simulink model "ART_IDS_TUNING_SLDRT"  (R2021a)
settings: configuration reference "Normal_SLDRT" (kept outside this file)
undefined symbols (not defined in the file): channel, group_IP_address, receive_multicast_udp_port_initialize, release_receive_multicast_udp_buffer, TRDP_COM_ID_CCU2IDS, TRDP_COM_ID_MC1_IDS2CCU, TRDP_COM_ID_MC1_MMU2IDS_POINT, TRDP_COM_ID_MC1_MMU2IDS_SEGMENT, TRDP_COM_ID_MC2_IDS2CCU, TRDP_COM_ID_MC2_MMU2IDS_POINT, TRDP_COM_ID_MC2_MMU2IDS_SEGMENT, TRDP_CONFIG_MC1_CCU2IDS, TRDP_CONFIG_MC1_IDS2CCU, TRDP_CONFIG_MC1_MMU2IDS_POINT, TRDP_CONFIG_MC1_MMU2IDS_SEGMENT, TRDP_CONFIG_MC2_CCU2IDS, TRDP_CONFIG_MC2_IDS2CCU, TRDP_CONFIG_MC2_MMU2IDS_POINT, TRDP_CONFIG_MC2_MMU2IDS_SEGMENT, TRDP_SIGNALS_MC1_CCU2IDS, TRDP_SIGNALS_MC1_IDS2CCU, TRDP_SIGNALS_MC1_MMU2IDS_POINT, TRDP_SIGNALS_MC1_MMU2IDS_SEGMENT, TRDP_SIGNALS_MC2_CCU2IDS, TRDP_SIGNALS_MC2_IDS2CCU, TRDP_SIGNALS_MC2_MMU2IDS_POINT, TRDP_SIGNALS_MC2_MMU2IDS_SEGMENT, UDP_port
libraries: simulink x1, sldrtlib x1
settings Model: DataDictionary=ART_IDS_TUNING.sldd  Creator=xinrui  LastModifiedBy=xinrui
settings ConfigSetRef: SourceName=Normal_SLDRT

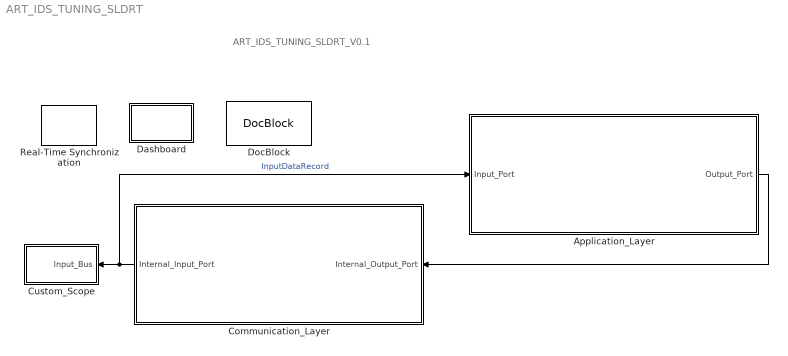
== system ART_IDS_TUNING_SLDRT ==
  note: ART_IDS_TUNING_SLDRT_V0.1
  Application_Layer : Subsystem
  Communication_Layer : Subsystem
  Custom_Scope : Subsystem
  Dashboard : Subsystem
  DocBlock : simulink/Model-Wide Utilities/DocBlock  DocumentType=HTML  mask(DocBlock){}
      mask Display:
      | plot([.8 0 0 1 1 .8 .8 1],[1 1 0 0 .8 1 .8 .8]);
      | text(.5,.6,'CHANGELOG','horizontalalignment','center');
      | text(.95,.05,get_param(gcb,'DocumentType'),'verticalalignment','bottom','horizontalalignment','right');
  Real-Time Synchronization : sldrtlib/Real-Time Synchronization  SampleTime=-1  MaxMissedTicks=100  ShowMissedTicks=off  YieldWhenWaiting=off
  wires:
  Application_Layer/1(Output_Port) -> Communication_Layer/1(Internal_Output_Port)
  Communication_Layer/1(Internal_Input_Port) -> Custom_Scope/1(Input_Bus), Application_Layer/1(Input_Port)  "InputDataRecord"

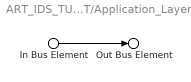
== system ART_IDS_TUNING_SLDRT/Application_Layer ==
  In Bus Element : Inport  PortName=Input_Port
  Out Bus Element : Outport  PortName=Output_Port
  wires:
  In Bus Element/1 -> Out Bus Element/1

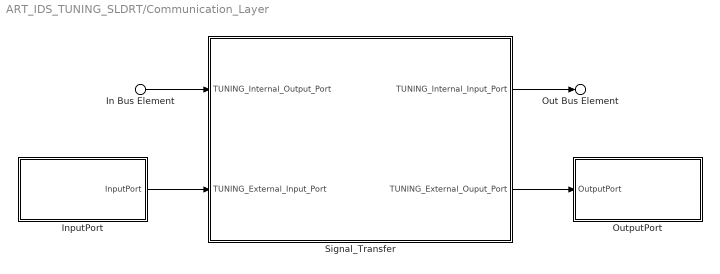
== system ART_IDS_TUNING_SLDRT/Communication_Layer ==
  In Bus Element : Inport  PortName=Internal_Output_Port
  InputPort : Subsystem
  OutputPort : Subsystem
  Signal_Transfer : Subsystem
  Out Bus Element : Outport  PortName=Internal_Input_Port
  wires:
  InputPort/1(InputPort) -> Signal_Transfer/2(TUNING_External_Input_Port)
  Signal_Transfer/2(TUNING_External_Ouput_Port) -> OutputPort/1(OutputPort)
  Signal_Transfer/1(TUNING_Internal_Input_Port) -> Out Bus Element/1
  In Bus Element/1 -> Signal_Transfer/1(TUNING_Internal_Output_Port)

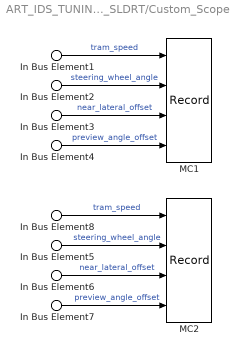
== system ART_IDS_TUNING_SLDRT/Custom_Scope ==
  In Bus Element2 : Inport  PortName=Input_Bus  Element=InputEthernet_bus.InputTRDP_bus.MC1_InputTRDP_bus.MC1_IDS2CCU_bus.SteeringWheelAngle
  In Bus Element3 : Inport  PortName=Input_Bus  Element=InputEthernet_bus.InputTRDP_bus.MC1_InputTRDP_bus.MC1_IDS2CCU_bus.NearLateralOffsetCurrent
  In Bus Element4 : Inport  PortName=Input_Bus  Element=InputEthernet_bus.InputTRDP_bus.MC1_InputTRDP_bus.MC1_IDS2CCU_bus.GNSSPreviewAngleOffset
  In Bus Element1 : Inport  PortName=Input_Bus  Element=InputEthernet_bus.InputTRDP_bus.MC1_InputTRDP_bus.MC1_CCU2IDS_bus.TramSpeed
  In Bus Element5 : Inport  PortName=Input_Bus  Element=InputEthernet_bus.InputTRDP_bus.MC2_InputTRDP_bus.MC2_IDS2CCU_bus.SteeringWheelAngle
  In Bus Element6 : Inport  PortName=Input_Bus  Element=InputEthernet_bus.InputTRDP_bus.MC2_InputTRDP_bus.MC2_IDS2CCU_bus.NearLateralOffsetCurrent
  In Bus Element7 : Inport  PortName=Input_Bus  Element=InputEthernet_bus.InputTRDP_bus.MC2_InputTRDP_bus.MC2_IDS2CCU_bus.GNSSPreviewAngleOffset
  In Bus Element8 : Inport  PortName=Input_Bus  Element=InputEthernet_bus.InputTRDP_bus.MC2_InputTRDP_bus.MC2_CCU2IDS_bus.TramSpeed
  MC1 : Record  FileSettingsInternal="{\"entries\":[{\"content\":{\"excelSettings\":{\"content\":{},\"type\":\"Streamout.ExcelSettings\"}},\"type\":\"Streamout.FileSettingStorage\",\"uuid\":\"18532c16-0af7-4887-b638-f8938ac9f1e5\"}],\"packageUris\":[\"http://schema.mathworks.com/mf0/streamout_blocks/R2020a\"],\"version\":\"1.0\"}"  Layout=[1 1]  SignalsInternal="{\"entries\":[{\"content\":{\"signals\":[{\"content\":{\"blockPath\":[\"ART_IDS_TUNING_SLDRT/Custom_Scope/MC1\"],\"channel\":[],\"dimensions\":[1],\"domain\":\"art_ids_tuning_sldrt/custom_scope/mc1\",\"lineColor\":\"#a2142f\",\"plots\":[1],\"port\":1,\"sid\":[\"\"],\"signalID\":17994,\"signalName\":\"tram_speed\"},\"type\":\"RecordBlkView.Signal\",\"uuid\":\"ffdbbce1-3832-4550-9eda-c42cbfad0fb4\"},{\"content\":{\"blockPath\":[\"ART_IDS_TUNING_SLDRT/Custom_Scope/MC1\"],\"channel\":[],\"dimensions\":[1],\"domain\":\"art_ids_tuning_sldrt/custom_scope/mc1\",\"lineColor\":\"#139fff\",\"plots\":[1],\"port\":2,\"sid\":[\"\"],\"signalID\":17998,\"signalName\":\"steering_wheel_angle\"},\"type\":\"RecordBlkView.Signal\",\"uuid\":\"9dfe40c3-a441-4cd7-9e23-c4ff49bc0eb6\"},{\"content\":{\"blockPath\":[\"ART_IDS_TUNING_SLDRT/Custom_Scope/MC1\"],\"channel\":[],\"dimensions\":[1],\"domain\":\"art_ids_tuning_sldrt/custom_scope/mc1\",\"lineColor\":\"#ff6929\",\"plots\":[1],\"port\":3,\"sid\":[\"\"],\"signalID\":18002,\"signalName\":\"near_lateral_offset\"},\"type\":\"RecordBlkView.Signal\",\"uuid\":\"35d5c813-d81d-4c05-befb-09d502742766\"},{\"content\":{\"blockPath\":[\"ART_IDS_TUNING_SLDRT/Custom_Scope/MC1\"],\"channel\":[],\"dimensions\":[1],\"domain\":\"art_ids_tuning_sldrt/custom_scope/mc1\",\"lineColor\":\"#b746ff\",\"plots\":[1],\"port\":4,\"sid\":[\"\"],\"signalID\":18006,\"signalName\":\"preview_angle_offset\"},\"type\":\"RecordBlkView.Signal\",\"uuid\":\"77379d0a-5e66-41a7-8f52-71aca193796f\"}]},\"type\":\"RecordBlkView.InputSignals\",\"uuid\":\"478cb186-bfdc-4c00-ad20-50ecaf964b6c\"}],\"packageUris\":[\"http://schema.mathworks.com/mf0/streamout_blocks/R2020a\"],\"version\":\"1.0\"}"  VisualizationBindings="{\"sparklinesplugin\":{\"info\":[{\"bindingParametersList\":[],\"subplotID\":1}]}}"
  MC2 : Record  FileSettingsInternal="{\"entries\":[{\"content\":{\"excelSettings\":{\"content\":{},\"type\":\"Streamout.ExcelSettings\"}},\"type\":\"Streamout.FileSettingStorage\",\"uuid\":\"80121879-a22b-4225-9770-3d7283b9ffe8\"}],\"packageUris\":[\"http://schema.mathworks.com/mf0/streamout_blocks/R2020a\"],\"version\":\"1.0\"}"  Layout=[1 1]  SignalsInternal="{\"entries\":[{\"content\":{\"signals\":[{\"content\":{\"blockPath\":[\"ART_IDS_TUNING_SLDRT/Custom_Scope/MC2\"],\"channel\":[],\"dimensions\":[1],\"domain\":\"art_ids_tuning_sldrt/custom_scope/mc2\",\"lineColor\":\"#64d413\",\"plots\":[1],\"port\":1,\"sid\":[\"\"],\"signalID\":18010,\"signalName\":\"tram_speed\"},\"type\":\"RecordBlkView.Signal\",\"uuid\":\"6fd8f2e4-7263-49d6-be86-0cf5ee5c4c70\"},{\"content\":{\"blockPath\":[\"ART_IDS_TUNING_SLDRT/Custom_Scope/MC2\"],\"channel\":[],\"dimensions\":[1],\"domain\":\"art_ids_tuning_sldrt/custom_scope/mc2\",\"lineColor\":\"#ff13a6\",\"plots\":[1],\"port\":2,\"sid\":[\"\"],\"signalID\":18014,\"signalName\":\"steering_wheel_angle\"},\"type\":\"RecordBlkView.Signal\",\"uuid\":\"65df261a-23f7-4e25-b953-a7d3bb80a214\"},{\"content\":{\"blockPath\":[\"ART_IDS_TUNING_SLDRT/Custom_Scope/MC2\"],\"channel\":[],\"dimensions\":[1],\"domain\":\"art_ids_tuning_sldrt/custom_scope/mc2\",\"lineColor\":\"#fe330a\",\"plots\":[1],\"port\":3,\"sid\":[\"\"],\"signalID\":18018,\"signalName\":\"near_lateral_offset\"},\"type\":\"RecordBlkView.Signal\",\"uuid\":\"bf99e8c5-f315-48f1-92bb-6e200dc516e7\"},{\"content\":{\"blockPath\":[\"ART_IDS_TUNING_SLDRT/Custom_Scope/MC2\"],\"channel\":[],\"dimensions\":[1],\"domain\":\"art_ids_tuning_sldrt/custom_scope/mc2\",\"lineColor\":\"#22b573\",\"plots\":[1],\"port\":4,\"sid\":[\"\"],\"signalID\":18022,\"signalName\":\"preview_angle_offset\"},\"type\":\"RecordBlkView.Signal\",\"uuid\":\"6624c94b-952c-48a7-9d72-709ee6e051d8\"}]},\"type\":\"RecordBlkView.InputSignals\",\"uuid\":\"f7d666a4-55db-46ce-8da9-48c4d2a57c10\"}],\"packageUris\":[\"http://schema.mathworks.com/mf0/streamout_blocks/R2020a\"],\"version\":\"1.0\"}"  VisualizationBindings="{\"sparklinesplugin\":{\"info\":[{\"bindingParametersList\":[],\"subplotID\":1}]}}"
  wires:
  In Bus Element1/1 -> MC1/1  "tram_speed"
  In Bus Element2/1 -> MC1/2  "steering_wheel_angle"
  In Bus Element3/1 -> MC1/3  "near_lateral_offset"
  In Bus Element4/1 -> MC1/4  "preview_angle_offset"
  In Bus Element7/1 -> MC2/4  "preview_angle_offset"
  In Bus Element6/1 -> MC2/3  "near_lateral_offset"
  In Bus Element5/1 -> MC2/2  "steering_wheel_angle"
  In Bus Element8/1 -> MC2/1  "tram_speed"

== system ART_IDS_TUNING_SLDRT/Dashboard ==

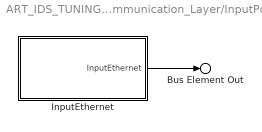
== system ART_IDS_TUNING_SLDRT/Communication_Layer/InputPort ==
  InputEthernet : Subsystem
  Bus Element Out : Outport  PortName=InputPort  Element=InputEthernet_bus
  wires:
  InputEthernet/1(InputEthernet) -> Bus Element Out/1

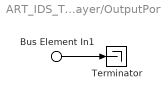
== system ART_IDS_TUNING_SLDRT/Communication_Layer/OutputPort ==
  Bus Element In1 : Inport  PortName=OutputPort
  Terminator : Terminator
  wires:
  Bus Element In1/1 -> Terminator/1

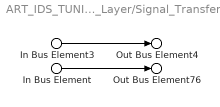
== system ART_IDS_TUNING_SLDRT/Communication_Layer/Signal_Transfer ==
  In Bus Element : Inport  PortName=TUNING_Internal_Output_Port
  In Bus Element3 : Inport  Port=2  PortName=TUNING_External_Input_Port
  Out Bus Element4 : Outport  PortName=TUNING_Internal_Input_Port
  Out Bus Element76 : Outport  Port=2  PortName=TUNING_External_Ouput_Port
  wires:
  In Bus Element/1 -> Out Bus Element76/1
  In Bus Element3/1 -> Out Bus Element4/1

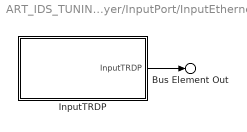
== system ART_IDS_TUNING_SLDRT/Communication_Layer/InputPort/InputEthernet ==
  InputTRDP : Subsystem
  Bus Element Out : Outport  PortName=InputEthernet  Element=InputTRDP_bus
  wires:
  InputTRDP/1(InputTRDP) -> Bus Element Out/1

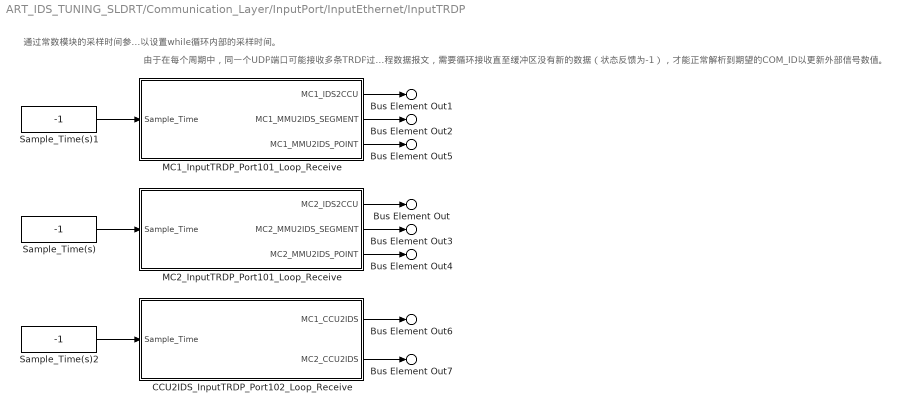
== system ART_IDS_TUNING_SLDRT/Communication_Layer/InputPort/InputEthernet/InputTRDP ==
  note: 通过常数模块的采样时间参数可以设置while循环内部的采样时间。
  note: 由于在每个周期中，同一个UDP端口可能接收多条TRDP过程数据报文，需要循环接收直至缓冲区没有新的数据（状态反馈为-1），才能正常解析到期望的COM_ID以更新外部信号数值。
  CCU2IDS_InputTRDP_Port102_Loop_Receive : Subsystem  TreatAsAtomicUnit=on
  MC1_InputTRDP_Port101_Loop_Receive : Subsystem  TreatAsAtomicUnit=on
  MC2_InputTRDP_Port101_Loop_Receive : Subsystem  TreatAsAtomicUnit=on
  Sample_Time(s) : Constant  Value=-1  SampleTime=-1
  Sample_Time(s)1 : Constant  Value=-1  SampleTime=-1
  Sample_Time(s)2 : Constant  Value=-1  SampleTime=-1
  Bus Element Out1 : Outport  PortName=InputTRDP  Element=MC1_InputTRDP_bus.MC1_IDS2CCU_bus
  Bus Element Out6 : Outport  PortName=InputTRDP  Element=MC1_InputTRDP_bus.MC1_CCU2IDS_bus
  Bus Element Out2 : Outport  PortName=InputTRDP  Element=MC1_InputTRDP_bus.MC1_MMU2IDS_SEGMENT_bus
  Bus Element Out5 : Outport  PortName=InputTRDP  Element=MC1_InputTRDP_bus.MC1_MMU2IDS_POINT_bus
  Bus Element Out : Outport  PortName=InputTRDP  Element=MC2_InputTRDP_bus.MC2_IDS2CCU_bus
  Bus Element Out7 : Outport  PortName=InputTRDP  Element=MC2_InputTRDP_bus.MC2_CCU2IDS_bus
  Bus Element Out3 : Outport  PortName=InputTRDP  Element=MC2_InputTRDP_bus.MC2_MMU2IDS_SEGMENT_bus
  Bus Element Out4 : Outport  PortName=InputTRDP  Element=MC2_InputTRDP_bus.MC2_MMU2IDS_POINT_bus
  wires:
  MC2_InputTRDP_Port101_Loop_Receive/1(MC2_IDS2CCU) -> Bus Element Out/1
  MC1_InputTRDP_Port101_Loop_Receive/2(MC1_MMU2IDS_SEGMENT) -> Bus Element Out2/1
  MC1_InputTRDP_Port101_Loop_Receive/1(MC1_IDS2CCU) -> Bus Element Out1/1
  MC2_InputTRDP_Port101_Loop_Receive/2(MC2_MMU2IDS_SEGMENT) -> Bus Element Out3/1
  Sample_Time(s)/1 -> MC2_InputTRDP_Port101_Loop_Receive/1(Sample_Time)
  MC1_InputTRDP_Port101_Loop_Receive/3(MC1_MMU2IDS_POINT) -> Bus Element Out5/1
  MC2_InputTRDP_Port101_Loop_Receive/3(MC2_MMU2IDS_POINT) -> Bus Element Out4/1
  Sample_Time(s)1/1 -> MC1_InputTRDP_Port101_Loop_Receive/1(Sample_Time)
  Sample_Time(s)2/1 -> CCU2IDS_InputTRDP_Port102_Loop_Receive/1(Sample_Time)
  CCU2IDS_InputTRDP_Port102_Loop_Receive/1(MC1_CCU2IDS) -> Bus Element Out6/1
  CCU2IDS_InputTRDP_Port102_Loop_Receive/2(MC2_CCU2IDS) -> Bus Element Out7/1

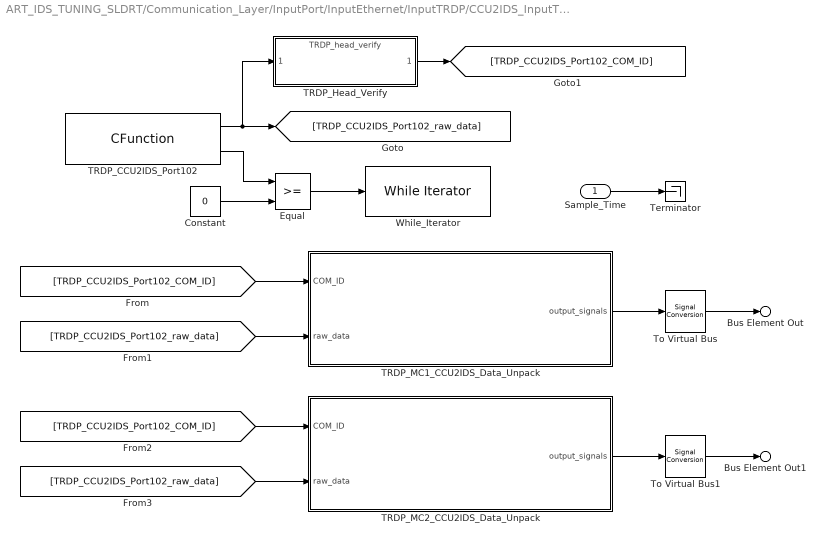
== system ART_IDS_TUNING_SLDRT/Communication_Layer/InputPort/InputEthernet/InputTRDP/CCU2IDS_InputTRDP_Port102_Loop_Receive ==
  Sample_Time : Inport
  Constant : Constant  Value=0  OutDataTypeStr=int32
  Equal : RelationalOperator  OutDataTypeStr=boolean  RndMeth=Simplest
  TRDP_CCU2IDS_Port102 : CFunction  OutputCode=|  TerminateCode=release_receive_multicast_udp_buffer(channel);  StartCode=receive_multicast_udp_port_initialize(group_IP_address, UDP_port, channel);  group_IP_address=uint8(['239.255.1.102',0])  UDP_port=int32(17224)  channel=int32(2)
      | int index;
      | uint8_T *receive_buffer;
      | data_length = receive_multicast_udp_data(channel);
      | receive_buffer = get_multicast_udp_data(channel);
      | for(index = 0; index < RECEIVE_MULTICAST_UDP_BUFFER_SIZE; index++)
      | {
      |     TRDP_input[index] = receive_buffer[index];
      | }
  TRDP_Head_Verify : ModelReference  ModelNameDialog=TRDP_head_verify  SimulationMode=Normal  ModelReferenceVersion=1.47
  TRDP_MC1_CCU2IDS_Data_Unpack : MATLAB Function  TreatAsAtomicUnit=on
  TRDP_MC2_CCU2IDS_Data_Unpack : MATLAB Function  TreatAsAtomicUnit=on
  Terminator : Terminator
  To Virtual Bus : SignalConversion  ConversionOutput=Virtual bus  OverrideOpt=off
  To Virtual Bus1 : SignalConversion  ConversionOutput=Virtual bus  OverrideOpt=off
  While_Iterator : WhileIterator  MaxIters=-1  WhileBlockType=do-while
  Bus Element Out : Outport  PortName=MC1_CCU2IDS
  Bus Element Out1 : Outport  Port=2  PortName=MC2_CCU2IDS
  wires:
  [TRDP_CCU2IDS_Port102_raw_data] -> TRDP_MC2_CCU2IDS_Data_Unpack/2(raw_data)
  [TRDP_CCU2IDS_Port102_COM_ID] -> TRDP_MC1_CCU2IDS_Data_Unpack/1(COM_ID)
  [TRDP_CCU2IDS_Port102_raw_data] -> TRDP_MC1_CCU2IDS_Data_Unpack/2(raw_data)
  TRDP_Head_Verify/1 -> [TRDP_CCU2IDS_Port102_COM_ID]
  To Virtual Bus1/1 -> Bus Element Out1/1
  TRDP_MC2_CCU2IDS_Data_Unpack/1(output_signals) -> To Virtual Bus1/1
  [TRDP_CCU2IDS_Port102_COM_ID] -> TRDP_MC2_CCU2IDS_Data_Unpack/1(COM_ID)
  TRDP_CCU2IDS_Port102/1 -> [TRDP_CCU2IDS_Port102_raw_data], TRDP_Head_Verify/1
  TRDP_CCU2IDS_Port102/2 -> Equal/1
  Constant/1 -> Equal/2
  TRDP_MC1_CCU2IDS_Data_Unpack/1(output_signals) -> To Virtual Bus/1
  To Virtual Bus/1 -> Bus Element Out/1
  Sample_Time/1 -> Terminator/1
  Equal/1 -> While_Iterator/1

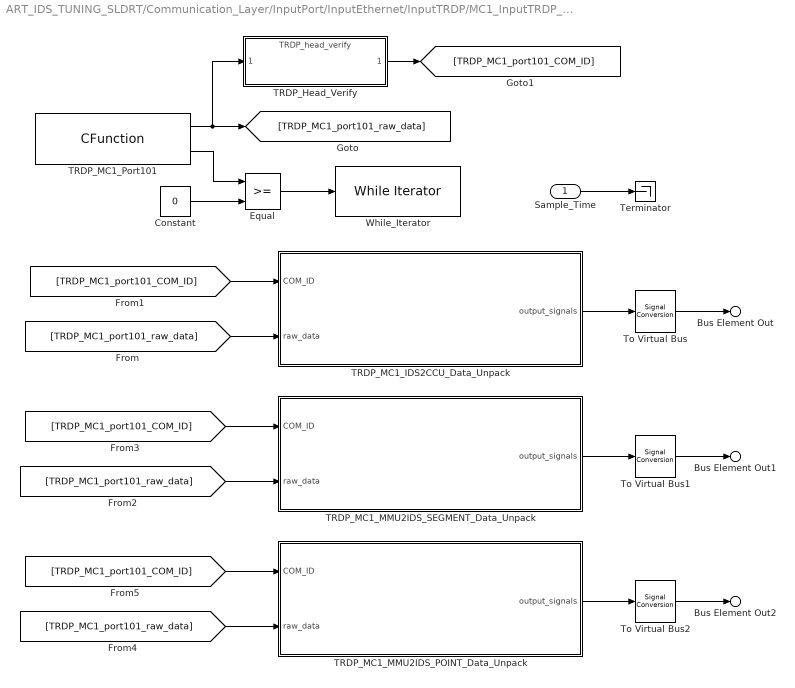
== system ART_IDS_TUNING_SLDRT/Communication_Layer/InputPort/InputEthernet/InputTRDP/MC1_InputTRDP_Port101_Loop_Receive ==
  Sample_Time : Inport
  Constant : Constant  Value=0  OutDataTypeStr=int32
  Equal : RelationalOperator  OutDataTypeStr=boolean  RndMeth=Simplest
  TRDP_Head_Verify : ModelReference  ModelNameDialog=TRDP_head_verify  SimulationMode=Normal  ModelReferenceVersion=1.47
  TRDP_MC1_IDS2CCU_Data_Unpack : MATLAB Function  TreatAsAtomicUnit=on
  TRDP_MC1_MMU2IDS_POINT_Data_Unpack : MATLAB Function  TreatAsAtomicUnit=on
  TRDP_MC1_MMU2IDS_SEGMENT_Data_Unpack : MATLAB Function  TreatAsAtomicUnit=on
  TRDP_MC1_Port101 : CFunction  OutputCode=|  TerminateCode=release_receive_multicast_udp_buffer(channel);  StartCode=receive_multicast_udp_port_initialize(group_IP_address, UDP_port, channel);  group_IP_address=uint8(['239.255.1.101',0])  UDP_port=int32(17224)  channel=int32(1)
      | int index;
      | uint8_T *receive_buffer;
      | data_length = receive_multicast_udp_data(channel);
      | receive_buffer = get_multicast_udp_data(channel);
      | for(index = 0; index < RECEIVE_MULTICAST_UDP_BUFFER_SIZE; index++)
      | {
      |     TRDP_input[index] = receive_buffer[index];
      | }
  Terminator : Terminator
  To Virtual Bus : SignalConversion  ConversionOutput=Virtual bus  OverrideOpt=off
  To Virtual Bus1 : SignalConversion  ConversionOutput=Virtual bus  OverrideOpt=off
  To Virtual Bus2 : SignalConversion  ConversionOutput=Virtual bus  OverrideOpt=off
  While_Iterator : WhileIterator  MaxIters=-1  WhileBlockType=do-while
  Bus Element Out : Outport  PortName=MC1_IDS2CCU
  Bus Element Out1 : Outport  Port=2  PortName=MC1_MMU2IDS_SEGMENT
  Bus Element Out2 : Outport  Port=3  PortName=MC1_MMU2IDS_POINT
  wires:
  [TRDP_MC1_port101_COM_ID] -> TRDP_MC1_MMU2IDS_POINT_Data_Unpack/1(COM_ID)
  TRDP_MC1_MMU2IDS_POINT_Data_Unpack/1(output_signals) -> To Virtual Bus2/1
  To Virtual Bus2/1 -> Bus Element Out2/1
  [TRDP_MC1_port101_raw_data] -> TRDP_MC1_MMU2IDS_POINT_Data_Unpack/2(raw_data)
  [TRDP_MC1_port101_raw_data] -> TRDP_MC1_MMU2IDS_SEGMENT_Data_Unpack/2(raw_data)
  [TRDP_MC1_port101_COM_ID] -> TRDP_MC1_IDS2CCU_Data_Unpack/1(COM_ID)
  [TRDP_MC1_port101_raw_data] -> TRDP_MC1_IDS2CCU_Data_Unpack/2(raw_data)
  TRDP_Head_Verify/1 -> [TRDP_MC1_port101_COM_ID]
  To Virtual Bus1/1 -> Bus Element Out1/1
  TRDP_MC1_MMU2IDS_SEGMENT_Data_Unpack/1(output_signals) -> To Virtual Bus1/1
  [TRDP_MC1_port101_COM_ID] -> TRDP_MC1_MMU2IDS_SEGMENT_Data_Unpack/1(COM_ID)
  TRDP_MC1_Port101/1 -> [TRDP_MC1_port101_raw_data], TRDP_Head_Verify/1
  TRDP_MC1_Port101/2 -> Equal/1
  Constant/1 -> Equal/2
  TRDP_MC1_IDS2CCU_Data_Unpack/1(output_signals) -> To Virtual Bus/1
  To Virtual Bus/1 -> Bus Element Out/1
  Sample_Time/1 -> Terminator/1
  Equal/1 -> While_Iterator/1

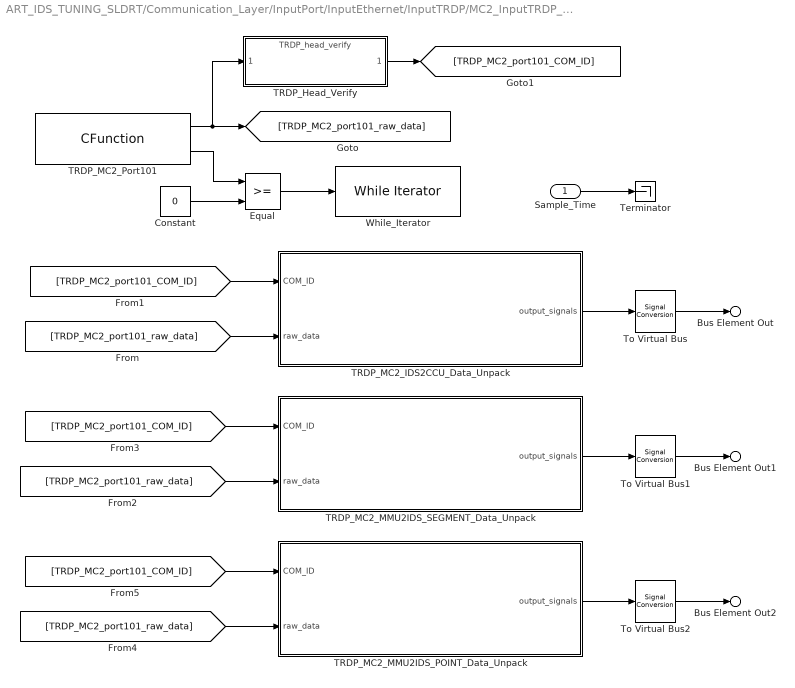
== system ART_IDS_TUNING_SLDRT/Communication_Layer/InputPort/InputEthernet/InputTRDP/MC2_InputTRDP_Port101_Loop_Receive ==
  Sample_Time : Inport
  Constant : Constant  Value=0  OutDataTypeStr=int32
  Equal : RelationalOperator  OutDataTypeStr=boolean  RndMeth=Simplest
  TRDP_Head_Verify : ModelReference  ModelNameDialog=TRDP_head_verify  SimulationMode=Normal  ModelReferenceVersion=1.47
  TRDP_MC2_IDS2CCU_Data_Unpack : MATLAB Function  TreatAsAtomicUnit=on
  TRDP_MC2_MMU2IDS_POINT_Data_Unpack : MATLAB Function  TreatAsAtomicUnit=on
  TRDP_MC2_MMU2IDS_SEGMENT_Data_Unpack : MATLAB Function  TreatAsAtomicUnit=on
  TRDP_MC2_Port101 : CFunction  OutputCode=|  TerminateCode=release_receive_multicast_udp_buffer(channel);  StartCode=receive_multicast_udp_port_initialize(group_IP_address, UDP_port, channel);  group_IP_address=uint8(['239.255.3.101',0])  UDP_port=int32(17224)  channel=int32(0)
      | int index;
      | uint8_T *receive_buffer;
      | data_length = receive_multicast_udp_data(channel);
      | receive_buffer = get_multicast_udp_data(channel);
      | for(index = 0; index < RECEIVE_MULTICAST_UDP_BUFFER_SIZE; index++)
      | {
      |     TRDP_input[index] = receive_buffer[index];
      | }
  Terminator : Terminator
  To Virtual Bus : SignalConversion  ConversionOutput=Virtual bus  OverrideOpt=off
  To Virtual Bus1 : SignalConversion  ConversionOutput=Virtual bus  OverrideOpt=off
  To Virtual Bus2 : SignalConversion  ConversionOutput=Virtual bus  OverrideOpt=off
  While_Iterator : WhileIterator  MaxIters=-1  WhileBlockType=do-while
  Bus Element Out : Outport  PortName=MC2_IDS2CCU
  Bus Element Out1 : Outport  Port=2  PortName=MC2_MMU2IDS_SEGMENT
  Bus Element Out2 : Outport  Port=3  PortName=MC2_MMU2IDS_POINT
  wires:
  Equal/1 -> While_Iterator/1
  Sample_Time/1 -> Terminator/1
  To Virtual Bus/1 -> Bus Element Out/1
  TRDP_MC2_IDS2CCU_Data_Unpack/1(output_signals) -> To Virtual Bus/1
  Constant/1 -> Equal/2
  TRDP_MC2_Port101/2 -> Equal/1
  TRDP_MC2_Port101/1 -> TRDP_Head_Verify/1, [TRDP_MC2_port101_raw_data]
  [TRDP_MC2_port101_COM_ID] -> TRDP_MC2_MMU2IDS_SEGMENT_Data_Unpack/1(COM_ID)
  TRDP_MC2_MMU2IDS_SEGMENT_Data_Unpack/1(output_signals) -> To Virtual Bus1/1
  To Virtual Bus1/1 -> Bus Element Out1/1
  TRDP_Head_Verify/1 -> [TRDP_MC2_port101_COM_ID]
  [TRDP_MC2_port101_raw_data] -> TRDP_MC2_IDS2CCU_Data_Unpack/2(raw_data)
  [TRDP_MC2_port101_COM_ID] -> TRDP_MC2_IDS2CCU_Data_Unpack/1(COM_ID)
  [TRDP_MC2_port101_raw_data] -> TRDP_MC2_MMU2IDS_SEGMENT_Data_Unpack/2(raw_data)
  [TRDP_MC2_port101_raw_data] -> TRDP_MC2_MMU2IDS_POINT_Data_Unpack/2(raw_data)
  To Virtual Bus2/1 -> Bus Element Out2/1
  TRDP_MC2_MMU2IDS_POINT_Data_Unpack/1(output_signals) -> To Virtual Bus2/1
  [TRDP_MC2_port101_COM_ID] -> TRDP_MC2_MMU2IDS_POINT_Data_Unpack/1(COM_ID)

== matlab function ART_IDS_TUNING_SLDRT/Communication_Layer/InputPort/InputEthernet/InputTRDP/CCU2IDS_InputTRDP_Port102_Loop_Receive/TRDP_MC2_CCU2IDS_Data_Unpack ==
  data: COM_ID input uint32 size=1; raw_data input uint8 size=1040; output_signals output Bus: MC2_CCU2IDS size=1; TRDP_CONFIG_MC2_CCU2IDS parameter Bus: CONFIG_MC2_CCU2IDS size=1; TRDP_SIGNALS_MC2_CCU2IDS parameter Bus: MC2_CCU2IDS size=1; TRDP_COM_ID_CCU2IDS parameter double size=1
% TRDP数据解包
function output_signals = TRDP_MC2_CCU2IDS_data_unpack(COM_ID, raw_data, ...
    TRDP_CONFIG_MC2_CCU2IDS, TRDP_SIGNALS_MC2_CCU2IDS, TRDP_COM_ID_CCU2IDS)
%   1.输入参数：
%       (1)COM_ID                      TRDP通信索引，1×1的uint32向量
%       (2)raw_data                    TRDP原始数据，1040×1的uint8向量
%       (3)TRDP_CONFIG_MC2_CCU2IDS     MC2端CCU发给IDS的TRDP原始数据解析配置参数，Parameter，数据字典中的一个结构体
%       (4)TRDP_SIGNALS_MC2_CCU2IDS    MC2端CCU发给IDS的TRDP信号结构初始值，Parameter，数据字典中的一个结构体
%       (5)TRDP_COM_ID_CCU2IDS         CCU发给IDS的TRDP过程数据COM ID，Parameter，数据字典中的一个Parameter变量
%   2.输出参数：
%       (1)output_signals              输出信号结构体，匹配MC2_CCU2IDS总线类型

%% 静态变量声明及初始化
% CCU2IDS信号结构体，用于存储上周期IDS相关信号数值
persistent TRDP_CCU2IDS_signals;
if isempty(TRDP_CCU2IDS_signals)
   TRDP_CCU2IDS_signals = TRDP_SIGNALS_MC2_CCU2IDS;
end

%% 检查COM_ID和数据长度，与预期匹配才则将后1000个字节解析为CCU2IDS数据
if TRDP_COM_ID_CCU2IDS == COM_ID && 1040 == length(raw_data)
    TRDP_CCU2IDS_signals = TRDP_input_data_parse(raw_data(41 : 1040), ...
        TRDP_CONFIG_MC2_CCU2IDS, TRDP_CCU2IDS_signals);
end

%% 输出信号赋值
output_signals = TRDP_CCU2IDS_signals;

end

== matlab function ART_IDS_TUNING_SLDRT/Communication_Layer/InputPort/InputEthernet/InputTRDP/MC2_InputTRDP_Port101_Loop_Receive/TRDP_MC2_MMU2IDS_SEGMENT_Data_Unpack ==
  data: COM_ID input uint32 size=1; raw_data input uint8 size=1040; output_signals output Bus: MC2_MMU2IDS_SEGMENT size=1; TRDP_CONFIG_MC2_MMU2IDS_SEGMENT parameter Bus: CONFIG_MC2_MMU2IDS_SEGMENT size=1; TRDP_SIGNALS_MC2_MMU2IDS_SEGMENT parameter Bus: MC2_MMU2IDS_SEGMENT size=1; TRDP_COM_ID_MC2_MMU2IDS_SEGMENT parameter double size=1
% TRDP数据解包
function output_signals = TRDP_MC2_MMU2IDS_SEGMENT_data_unpack(COM_ID, raw_data, ...
    TRDP_CONFIG_MC2_MMU2IDS_SEGMENT, TRDP_SIGNALS_MC2_MMU2IDS_SEGMENT, ...
    TRDP_COM_ID_MC2_MMU2IDS_SEGMENT)
%   1.输入参数：
%       (1)COM_ID                              TRDP通信索引，1×1的uint32向量
%       (2)raw_data                            TRDP原始数据，1040×1的uint8向量
%       (3)TRDP_CONFIG_MC2_MMU2IDS_SEGMENT     MC2端MMU发给IDS的区间配置TRDP原始数据解析配置参数，Parameter，数据字典中的一个结构体
%       (4)TRDP_SIGNALS_MC2_MMU2IDS_SEGMENT    MC2端MMU发给IDS的区间配置TRDP信号结构初始值，Parameter，数据字典中的一个结构体
%       (5)TRDP_COM_ID_MC2_MMU2IDS_SEGMENT     MC2端MMU发给IDS的区间配置TRDP过程数据COM ID，Parameter，数据字典中的一个Parameter变量
%   2.输出参数：
%       (1)output_signals                      输出信号结构体，匹配MC2_MMU2IDS_SEGMENT总线类型

%% 静态变量声明及初始化
% MMU2IDS_SEGMENT信号结构体，用于存储上周期IDS相关信号数值
persistent TRDP_MMU2IDS_SEGMENT_signals;
if isempty(TRDP_MMU2IDS_SEGMENT_signals)
   TRDP_MMU2IDS_SEGMENT_signals = TRDP_SIGNALS_MC2_MMU2IDS_SEGMENT;
end

%% 检查COM_ID和数据长度，与预期匹配才则将后1000个字节解析为MMU2IDS_SEGMENT数据
if TRDP_COM_ID_MC2_MMU2IDS_SEGMENT == COM_ID && 1040 == length(raw_data)
    TRDP_MMU2IDS_SEGMENT_signals = TRDP_input_data_parse(raw_data(41 : 1040), ...
        TRDP_CONFIG_MC2_MMU2IDS_SEGMENT, TRDP_MMU2IDS_SEGMENT_signals);
end

%% 输出信号赋值
output_signals = TRDP_MMU2IDS_SEGMENT_signals;

end

== matlab function ART_IDS_TUNING_SLDRT/Communication_Layer/InputPort/InputEthernet/InputTRDP/MC2_InputTRDP_Port101_Loop_Receive/TRDP_MC2_MMU2IDS_POINT_Data_Unpack ==
  data: COM_ID input uint32 size=1; raw_data input uint8 size=1040; output_signals output Bus: MC2_MMU2IDS_POINT size=1; TRDP_CONFIG_MC2_MMU2IDS_POINT parameter Bus: CONFIG_MC2_MMU2IDS_POINT size=1; TRDP_SIGNALS_MC2_MMU2IDS_POINT parameter Bus: MC2_MMU2IDS_POINT size=1; TRDP_COM_ID_MC2_MMU2IDS_POINT parameter double size=1
% TRDP数据解包
function output_signals = TRDP_MC2_MMU2IDS_POINT_data_unpack(COM_ID, raw_data, ...
    TRDP_CONFIG_MC2_MMU2IDS_POINT, TRDP_SIGNALS_MC2_MMU2IDS_POINT, ...
    TRDP_COM_ID_MC2_MMU2IDS_POINT)
%   1.输入参数：
%       (1)COM_ID                            TRDP通信索引，1×1的uint32向量
%       (2)raw_data                          TRDP原始数据，1040×1的uint8向量
%       (3)TRDP_CONFIG_MC2_MMU2IDS_POINT     MC2端MMU发给IDS的轨迹属性TRDP原始数据解析配置参数，Parameter，数据字典中的一个结构体
%       (4)TRDP_SIGNALS_MC2_MMU2IDS_POINT    MC2端MMU发给IDS的轨迹属性TRDP信号结构初始值，Parameter，数据字典中的一个结构体
%       (5)TRDP_COM_ID_MC2_MMU2IDS_POINT     MC2端MMU发给IDS的轨迹属性TRDP过程数据COM ID，Parameter，数据字典中的一个Parameter变量
%   2.输出参数：
%       (1)output_signals                    输出信号结构体，匹配MC2_MMU2IDS_POINT总线类型

%% 静态变量声明及初始化
% MMU2IDS_POINT信号结构体，用于存储上周期IDS相关信号数值
persistent TRDP_MMU2IDS_POINT_signals;
if isempty(TRDP_MMU2IDS_POINT_signals)
   TRDP_MMU2IDS_POINT_signals = TRDP_SIGNALS_MC2_MMU2IDS_POINT;
end

%% 检查COM_ID和数据长度，与预期匹配才则将后1000个字节解析为MMU2IDS_POINT数据
if TRDP_COM_ID_MC2_MMU2IDS_POINT == COM_ID && 1040 == length(raw_data)
    TRDP_MMU2IDS_POINT_signals = TRDP_input_data_parse(raw_data(41 : 1040), ...
        TRDP_CONFIG_MC2_MMU2IDS_POINT, TRDP_MMU2IDS_POINT_signals);
end

%% 输出信号赋值
output_signals = TRDP_MMU2IDS_POINT_signals;

end

== matlab function ART_IDS_TUNING_SLDRT/Communication_Layer/InputPort/InputEthernet/InputTRDP/MC1_InputTRDP_Port101_Loop_Receive/TRDP_MC1_IDS2CCU_Data_Unpack ==
  data: COM_ID input uint32 size=1; raw_data input uint8 size=1040; output_signals output Bus: MC1_IDS2CCU size=1; TRDP_CONFIG_MC1_IDS2CCU parameter Bus: CONFIG_MC1_IDS2CCU size=1; TRDP_SIGNALS_MC1_IDS2CCU parameter Bus: MC1_IDS2CCU size=1; TRDP_COM_ID_MC1_IDS2CCU parameter double size=1
% TRDP数据解包
function output_signals = TRDP_MC1_IDS2CCU_data_unpack(COM_ID, raw_data, ...
    TRDP_CONFIG_MC1_IDS2CCU, TRDP_SIGNALS_MC1_IDS2CCU, TRDP_COM_ID_MC1_IDS2CCU)
%   1.输入参数：
%       (1)COM_ID                      TRDP通信索引，1×1的uint32向量
%       (2)raw_data                    TRDP原始数据，1040×1的uint8向量
%       (3)TRDP_CONFIG_MC1_IDS2CCU     MC1端IDS发给CCU的TRDP原始数据解析配置参数，Parameter，数据字典中的一个结构体
%       (4)TRDP_SIGNALS_MC1_IDS2CCU    MC1端IDS发给CCU的TRDP信号结构初始值，Parameter，数据字典中的一个结构体
%       (5)TRDP_COM_ID_MC1_IDS2CCU     MC1端IDS发给CCU的TRDP过程数据COM ID，Parameter，数据字典中的一个Parameter变量
%   2.输出参数：
%       (1)output_signals              输出信号结构体，匹配MC1_IDS2CCU总线类型

%% 静态变量声明及初始化
% IDS2CCU信号结构体，用于存储上周期IDS相关信号数值
persistent TRDP_IDS2CCU_signals;
if isempty(TRDP_IDS2CCU_signals)
   TRDP_IDS2CCU_signals = TRDP_SIGNALS_MC1_IDS2CCU;
end

%% 检查COM_ID和数据长度，与预期匹配才则将后1000个字节解析为IDS2CCU数据
if TRDP_COM_ID_MC1_IDS2CCU == COM_ID && 1040 == length(raw_data)
    TRDP_IDS2CCU_signals = TRDP_input_data_parse(raw_data(41 : 1040), ...
        TRDP_CONFIG_MC1_IDS2CCU, TRDP_IDS2CCU_signals);
end

%% 输出信号赋值
output_signals = TRDP_IDS2CCU_signals;

end

== matlab function ART_IDS_TUNING_SLDRT/Communication_Layer/InputPort/InputEthernet/InputTRDP/MC2_InputTRDP_Port101_Loop_Receive/TRDP_MC2_IDS2CCU_Data_Unpack ==
  data: COM_ID input uint32 size=1; raw_data input uint8 size=1040; output_signals output Bus: MC2_IDS2CCU size=1; TRDP_CONFIG_MC2_IDS2CCU parameter Bus: CONFIG_MC2_IDS2CCU size=1; TRDP_SIGNALS_MC2_IDS2CCU parameter Bus: MC2_IDS2CCU size=1; TRDP_COM_ID_MC2_IDS2CCU parameter double size=1
% TRDP数据解包
function output_signals = TRDP_MC2_IDS2CCU_data_unpack(COM_ID, raw_data, ...
    TRDP_CONFIG_MC2_IDS2CCU, TRDP_SIGNALS_MC2_IDS2CCU, TRDP_COM_ID_MC2_IDS2CCU)
%   1.输入参数：
%       (1)COM_ID                      TRDP通信索引，1×1的uint32向量
%       (2)raw_data                    TRDP原始数据，1040×1的uint8向量
%       (3)TRDP_CONFIG_MC2_IDS2CCU     MC2端IDS发给CCU的TRDP原始数据解析配置参数，Parameter，数据字典中的一个结构体
%       (4)TRDP_SIGNALS_MC2_IDS2CCU    MC2端IDS发给CCU的TRDP信号结构初始值，Parameter，数据字典中的一个结构体
%       (5)TRDP_COM_ID_MC2_IDS2CCU     MC2端IDS发给CCU的TRDP过程数据COM ID，Parameter，数据字典中的一个Parameter变量
%   2.输出参数：
%       (1)output_signals              输出信号结构体，匹配MC2_IDS2CCU总线类型

%% 静态变量声明及初始化
% IDS2CCU信号结构体，用于存储上周期IDS相关信号数值
persistent TRDP_IDS2CCU_signals;
if isempty(TRDP_IDS2CCU_signals)
   TRDP_IDS2CCU_signals = TRDP_SIGNALS_MC2_IDS2CCU;
end

%% 检查COM_ID和数据长度，与预期匹配才则将后1000个字节解析为IDS2CCU数据
if TRDP_COM_ID_MC2_IDS2CCU == COM_ID && 1040 == length(raw_data)
    TRDP_IDS2CCU_signals = TRDP_input_data_parse(raw_data(41 : 1040), ...
        TRDP_CONFIG_MC2_IDS2CCU, TRDP_IDS2CCU_signals);
end

%% 输出信号赋值
output_signals = TRDP_IDS2CCU_signals;

end

== matlab function ART_IDS_TUNING_SLDRT/Communication_Layer/InputPort/InputEthernet/InputTRDP/MC1_InputTRDP_Port101_Loop_Receive/TRDP_MC1_MMU2IDS_POINT_Data_Unpack ==
  data: COM_ID input uint32 size=1; raw_data input uint8 size=1040; output_signals output Bus: MC1_MMU2IDS_POINT size=1; TRDP_CONFIG_MC1_MMU2IDS_POINT parameter Bus: CONFIG_MC1_MMU2IDS_POINT size=1; TRDP_SIGNALS_MC1_MMU2IDS_POINT parameter Bus: MC1_MMU2IDS_POINT size=1; TRDP_COM_ID_MC1_MMU2IDS_POINT parameter double size=1
% TRDP数据解包
function output_signals = TRDP_MC1_MMU2IDS_POINT_data_unpack(COM_ID, raw_data, ...
    TRDP_CONFIG_MC1_MMU2IDS_POINT, TRDP_SIGNALS_MC1_MMU2IDS_POINT, ...
    TRDP_COM_ID_MC1_MMU2IDS_POINT)
%   1.输入参数：
%       (1)COM_ID                            TRDP通信索引，1×1的uint32向量
%       (2)raw_data                          TRDP原始数据，1040×1的uint8向量
%       (3)TRDP_CONFIG_MC1_MMU2IDS_POINT     MC1端MMU发给IDS的轨迹属性TRDP原始数据解析配置参数，Parameter，数据字典中的一个结构体
%       (4)TRDP_SIGNALS_MC1_MMU2IDS_POINT    MC1端MMU发给IDS的轨迹属性TRDP信号结构初始值，Parameter，数据字典中的一个结构体
%       (5)TRDP_COM_ID_MC1_MMU2IDS_POINT     MC1端MMU发给IDS的轨迹属性TRDP过程数据COM ID，Parameter，数据字典中的一个Parameter变量
%   2.输出参数：
%       (1)output_signals                    输出信号结构体，匹配MC1_MMU2IDS_POINT总线类型

%% 静态变量声明及初始化
% MMU2IDS_POINT信号结构体，用于存储上周期IDS相关信号数值
persistent TRDP_MMU2IDS_POINT_signals;
if isempty(TRDP_MMU2IDS_POINT_signals)
   TRDP_MMU2IDS_POINT_signals = TRDP_SIGNALS_MC1_MMU2IDS_POINT;
end

%% 检查COM_ID和数据长度，与预期匹配才则将后1000个字节解析为MMU2IDS_POINT数据
if TRDP_COM_ID_MC1_MMU2IDS_POINT == COM_ID && 1040 == length(raw_data)
    TRDP_MMU2IDS_POINT_signals = TRDP_input_data_parse(raw_data(41 : 1040), ...
        TRDP_CONFIG_MC1_MMU2IDS_POINT, TRDP_MMU2IDS_POINT_signals);
end

%% 输出信号赋值
output_signals = TRDP_MMU2IDS_POINT_signals;

end

== matlab function ART_IDS_TUNING_SLDRT/Communication_Layer/InputPort/InputEthernet/InputTRDP/MC1_InputTRDP_Port101_Loop_Receive/TRDP_MC1_MMU2IDS_SEGMENT_Data_Unpack ==
  data: COM_ID input uint32 size=1; raw_data input uint8 size=1040; output_signals output Bus: MC1_MMU2IDS_SEGMENT size=1; TRDP_CONFIG_MC1_MMU2IDS_SEGMENT parameter Bus: CONFIG_MC1_MMU2IDS_SEGMENT size=1; TRDP_SIGNALS_MC1_MMU2IDS_SEGMENT parameter Bus: MC1_MMU2IDS_SEGMENT size=1; TRDP_COM_ID_MC1_MMU2IDS_SEGMENT parameter double size=1
% TRDP数据解包
function output_signals = TRDP_MC1_MMU2IDS_SEGMENT_data_unpack(COM_ID, raw_data, ...
    TRDP_CONFIG_MC1_MMU2IDS_SEGMENT, TRDP_SIGNALS_MC1_MMU2IDS_SEGMENT, ...
    TRDP_COM_ID_MC1_MMU2IDS_SEGMENT)
%   1.输入参数：
%       (1)COM_ID                              TRDP通信索引，1×1的uint32向量
%       (2)raw_data                            TRDP原始数据，1040×1的uint8向量
%       (3)TRDP_CONFIG_MC1_MMU2IDS_SEGMENT     MC1端MMU发给IDS的区间配置TRDP原始数据解析配置参数，Parameter，数据字典中的一个结构体
%       (4)TRDP_SIGNALS_MC1_MMU2IDS_SEGMENT    MC1端MMU发给IDS的区间配置TRDP信号结构初始值，Parameter，数据字典中的一个结构体
%       (5)TRDP_COM_ID_MC1_MMU2IDS_SEGMENT     MC1端MMU发给IDS的区间配置TRDP过程数据COM ID，Parameter，数据字典中的一个Parameter变量
%   2.输出参数：
%       (1)output_signals                      输出信号结构体，匹配MC1_MMU2IDS_SEGMENT总线类型

%% 静态变量声明及初始化
% MMU2IDS_SEGMENT信号结构体，用于存储上周期IDS相关信号数值
persistent TRDP_MMU2IDS_SEGMENT_signals;
if isempty(TRDP_MMU2IDS_SEGMENT_signals)
   TRDP_MMU2IDS_SEGMENT_signals = TRDP_SIGNALS_MC1_MMU2IDS_SEGMENT;
end

%% 检查COM_ID和数据长度，与预期匹配才则将后1000个字节解析为MMU2IDS_SEGMENT数据
if TRDP_COM_ID_MC1_MMU2IDS_SEGMENT == COM_ID && 1040 == length(raw_data)
    TRDP_MMU2IDS_SEGMENT_signals = TRDP_input_data_parse(raw_data(41 : 1040), ...
        TRDP_CONFIG_MC1_MMU2IDS_SEGMENT, TRDP_MMU2IDS_SEGMENT_signals);
end

%% 输出信号赋值
output_signals = TRDP_MMU2IDS_SEGMENT_signals;

end

== matlab function ART_IDS_TUNING_SLDRT/Communication_Layer/InputPort/InputEthernet/InputTRDP/CCU2IDS_InputTRDP_Port102_Loop_Receive/TRDP_MC1_CCU2IDS_Data_Unpack ==
  data: COM_ID input uint32 size=1; raw_data input uint8 size=1040; output_signals output Bus: MC1_CCU2IDS size=1; TRDP_CONFIG_MC1_CCU2IDS parameter Bus: CONFIG_MC1_CCU2IDS size=1; TRDP_SIGNALS_MC1_CCU2IDS parameter Bus: MC1_CCU2IDS size=1; TRDP_COM_ID_CCU2IDS parameter double size=1
% TRDP数据解包
function output_signals = TRDP_MC1_CCU2IDS_data_unpack(COM_ID, raw_data, ...
    TRDP_CONFIG_MC1_CCU2IDS, TRDP_SIGNALS_MC1_CCU2IDS, TRDP_COM_ID_CCU2IDS)
%   1.输入参数：
%       (1)COM_ID                      TRDP通信索引，1×1的uint32向量
%       (2)raw_data                    TRDP原始数据，1040×1的uint8向量
%       (3)TRDP_CONFIG_MC1_CCU2IDS     MC1端CCU发给IDS的TRDP原始数据解析配置参数，Parameter，数据字典中的一个结构体
%       (4)TRDP_SIGNALS_MC1_CCU2IDS    MC1端CCU发给IDS的TRDP信号结构初始值，Parameter，数据字典中的一个结构体
%       (5)TRDP_COM_ID_CCU2IDS         CCU发给IDS的TRDP过程数据COM ID，Parameter，数据字典中的一个Parameter变量
%   2.输出参数：
%       (1)output_signals              输出信号结构体，匹配MC1_CCU2IDS总线类型

%% 静态变量声明及初始化
% CCU2IDS信号结构体，用于存储上周期IDS相关信号数值
persistent TRDP_CCU2IDS_signals;
if isempty(TRDP_CCU2IDS_signals)
   TRDP_CCU2IDS_signals = TRDP_SIGNALS_MC1_CCU2IDS;
end

%% 检查COM_ID和数据长度，与预期匹配才则将后1000个字节解析为CCU2IDS数据
if TRDP_COM_ID_CCU2IDS == COM_ID && 1040 == length(raw_data)
    TRDP_CCU2IDS_signals = TRDP_input_data_parse(raw_data(41 : 1040), ...
        TRDP_CONFIG_MC1_CCU2IDS, TRDP_CCU2IDS_signals);
end

%% 输出信号赋值
output_signals = TRDP_CCU2IDS_signals;

end
